simulink model "run_c"  (R2024b)
settings: Solver=VariableStepAuto  StartTime=0.0  StopTime=10.0  RelTol=1e-3
values from neighbouring files (symbols this model uses):
  input_values = single(reshape(input(index,:), [dim_1, dim_2]))    [tf_to_c_mat.m]
  temp_max = 184.88    [tf_to_c_mat.m]
  temp_min = 19.6    [tf_to_c_mat.m]
libraries: deeplib x1
settings Model: Creator=dx5entre  LastModifiedBy=dx5entre
settings SFSimCC: SimCustomHeaderCode="# include \"models_matlab/Original/Predict0_ert_rtw/Predict0.h\""  SimUserSources=models_matlab/Original/Predict0_ert_rtw/Predict0.c

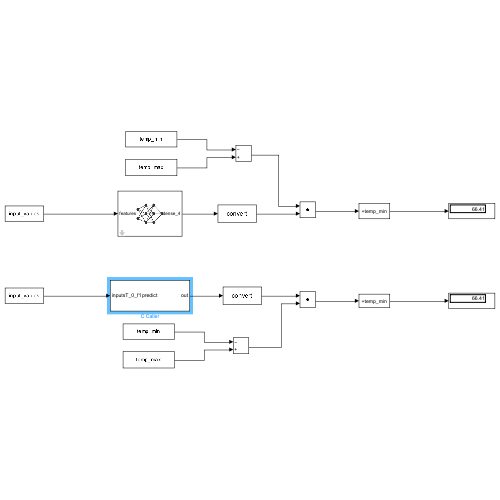
[thumbnail: Simulink's stored preview of the top-level diagram]
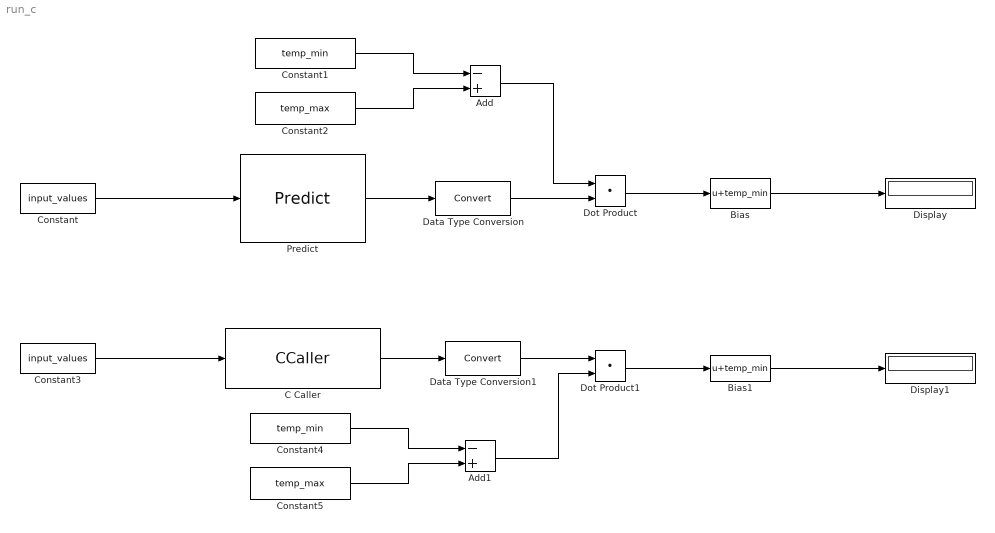
== system run_c ==
  Add : Sum  Inputs=-+
  Add1 : Sum  Inputs=-+
  Bias : Bias  Bias=temp_min  SaturateOnIntegerOverflow=off
  Bias1 : Bias  Bias=temp_min  SaturateOnIntegerOverflow=off
  C Caller : CCaller  FunctionName=predict  PortSpecificationStruct="%)30     .    V ,   8    (     @         %    \"     (    !     0         %  0 \"0    $    _    07)G3F%M90  4&]R=$YA;64 4V-O<&4     26YD97@     5'EP90      4VEZ90      27-';&]B86P   X    P    !@    @    $          4    (     0    ,    !         !   P!O=70 #@   #     &    \"     0         !0    @    !     P    $         $  # &]U=  .    .     8    (    !          %    \"     $    &     0         0    !@   $]U='!U=   #@   #@    &    \"     8         !0    @    !     0    $         \"0    @               X    X    !@    @    $          4    (     0    8    !         !     &    <VEN9VQE   .    ,     8    (    !          %    \"     $    !     0         0  $ ,0    X    P    !@    @    ) @        4    (     0    $    !          (  0      #@   $     &    \"     0         !0    @    !    #     $         $     P   !I;G!U='-47S!?9C$     #@   $     &    \"     0         !0    @    !    #     $         $     P   !I;G!U='-47S!?9C$     #@   #@    &    \"     0         !0    @    !    !0    $         $     4   !);G!U=     X    X    !@    @    &          4    (     0    $    !          D    (               .    .     8    (    !          %    \"     $    &     0         0    !@   '-I;F=L90  #@   #     &    \"     0         !0    @    !     @    $         $  \" #,U   .    ,     8    (    \"0(        %    \"     $    !     0         \"  $"
  Constant : Constant  Value=input_values  VectorParams1D=off
  Constant1 : Constant  Value=temp_min
  Constant2 : Constant  Value=temp_max
  Constant3 : Constant  Value=input_values  VectorParams1D=off
  Constant4 : Constant  Value=temp_min
  Constant5 : Constant  Value=temp_max
  Data Type Conversion : DataTypeConversion  SaturateOnIntegerOverflow=off  RndMeth=Floor
  Data Type Conversion1 : DataTypeConversion  SaturateOnIntegerOverflow=off  RndMeth=Floor
  Display : Display
  Display1 : Display
  Dot Product : DotProduct  OutDataTypeStr=Inherit: Inherit via internal rule
  Dot Product1 : DotProduct  OutDataTypeStr=Inherit: Inherit via internal rule
  Predict : deeplib/Predict  Network=Network from MAT-file  NetworkFunction=squeezenet  NetworkFilePath=C:\Users\dx5entre\Documents\Spang\edge-ai\Jupyter\models\Model_113_FCNN\Model_113_FCNN.mat  MiniBatchSize=128  InputDataFormats={ 'features', 'BC' }  Predictions=on  Activations={}  ForceInterpretedSim=off  EnableDLNetwork=on  LastKnownNetworkFilePath='C:\Users\dx5entre\Documents\Spang\edge-ai\Jupyter\models\Model_113_FCNN\Model_113_FCNN.mat'  LastKnownNetworkTimeStamp=739814.35143518517725169658660888671875
  wires:
  Constant1/1 -> Add/1
  Constant2/1 -> Add/2
  Predict/1 -> Data Type Conversion/1
  Data Type Conversion/1 -> Dot Product/2
  Dot Product/1 -> Bias/1
  Dot Product1/1 -> Bias1/1
  Bias/1 -> Display/1
  Bias1/1 -> Display1/1
  Constant/1 -> Predict/1
  Add/1 -> Dot Product/1
  Constant4/1 -> Add1/1
  Constant5/1 -> Add1/2
  Data Type Conversion1/1 -> Dot Product1/1
  Add1/1 -> Dot Product1/2
  C Caller/1 -> Data Type Conversion1/1
  Constant3/1 -> C Caller/1
